simulink model "nonlinear_ss"  (R2023b)
settings: Solver=VariableStepAuto  StartTime=0.0  StopTime=10.0  RelTol=1e-3
undefined symbols (not defined in the file or in its folder): a1, a2, a3, a4, a5, a6, control_switch, g1, g2, H, K, x_initial
settings Model: Creator=deniskirbaba  LastModifiedBy=deniskirbaba

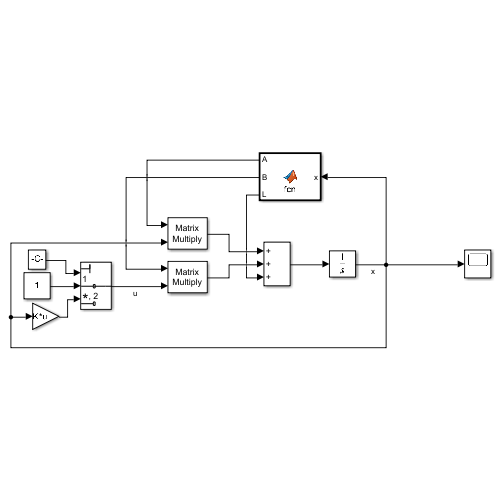
[thumbnail: Simulink's stored preview of the top-level diagram]
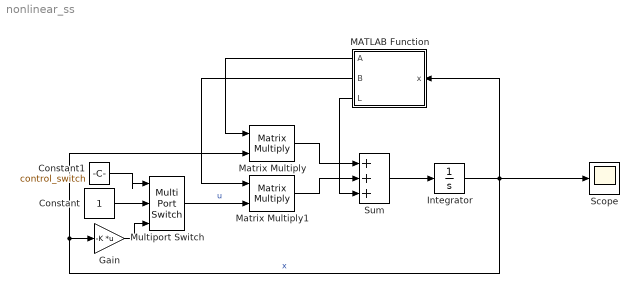
== system nonlinear_ss ==
  Constant : Constant
  Constant1 : Constant  Value=control_switch
  Gain : Gain  Gain=-K  Multiplication=Matrix(K*u)
  Integrator : Integrator  InitialCondition=x_initial
  MATLAB Function : MATLAB Function  TreatAsAtomicUnit=on
  Matrix Multiply : Product  Multiplication=Matrix(*)
  Matrix Multiply1 : Product  Multiplication=Matrix(*)
  Multiport Switch : MultiPortSwitch  Inputs=2  SaturateOnIntegerOverflow=off  InputSameDT=off
  Scope : Scope
  Sum : Sum  Inputs=+++
  wires:
  Sum/1 -> Integrator/1
  Integrator/1 -> Scope/1, Gain/1, Matrix Multiply/2, MATLAB Function/1(x)  "x"
  MATLAB Function/1(A) -> Matrix Multiply/1
  MATLAB Function/2(B) -> Matrix Multiply1/1
  MATLAB Function/3(L) -> Sum/3
  Matrix Multiply1/1 -> Sum/2
  Matrix Multiply/1 -> Sum/1
  Constant/1 -> Multiport Switch/2
  Multiport Switch/1 -> Matrix Multiply1/2  "u"
  Constant1/1 -> Multiport Switch/1
  Gain/1 -> Multiport Switch/3

== matlab function nonlinear_ss/MATLAB Function ==
  data: x input; A output size=[6, 6]; a1 parameter; a2 parameter; a3 parameter; a4 parameter; a5 parameter; a6 parameter; B output size=[6, 1]; L output size=[6, 1]; g1 parameter; g2 parameter; H parameter
function [A, B, L]= fcn(x, a1, a2, a3, a4, a5, a6, g1, g2, H)

M_inv = inv([a1 a2*cos(x(2)) a3*cos(x(3));
                 a2*cos(x(2)) a4 a5*cos(x(2)-x(3));
                 a3*cos(x(3)) a5*cos(x(2)-x(3)) a6]);
C = [0 -a2*sin(x(2))*x(5) -a3*sin(x(3))*x(6);
     0 0 a5*sin(x(2)-x(3))*x(6);
     0 -a5*sin(x(2)-x(3))*x(5) 0];
G = [0; -g1*sin(x(2)); -g2*sin(x(3))];

A = [zeros([3 3]), eye(3);
     zeros([3 3]), -M_inv*C];
B = [zeros([3 1]);
     M_inv*H];
L = [zeros([3 1]);
     -M_inv*G];
